simulink model "solarboat_solar"  (R2022a)
settings: Solver=VariableStepAuto  StartTime=0.0  StopTime=100  RelTol=1e-3
model workspace (MAT data in the model file):
  B = 0.67
  Cf = 0.00361699607356
  Dp = 0.2
  J = 1.6925
  K = 10
  KQ = 0.0168
  KT = 0.0514
  LOA = 1.8
  Re = 3577817.53131
  T = 1
  U = 5
  V_abs = 2
  d = 0.2
  mu = 1.188e-06
  psi_t = 0.174532925199
  rho = 1025
  weight = 8.036
  x_wp = 100
  y_wp = 100
libraries: fl_lib x12, nesl_utility x6, ee_lib x3, dspsrcs4 x2, slpidlib x1, spsPVArrayLib x1
settings Model: NumberOfSteps=100  Creator=takuya  LastModifiedBy=nakashima
settings OptimizationCC: ZeroExternalMemoryAtStartup=off  ZeroInternalMemoryAtStartup=off
settings DebuggingCC: UnconnectedInputMsg=warning  UnconnectedOutputMsg=warning  UnconnectedLineMsg=warning
settings RTWCC: TargetLang=C++  DLArmComputeVersion=19.05
settings GRTTargetCC: TargetLangStandard=C++11 (ISO)  CodeInterfacePackaging=C++ class

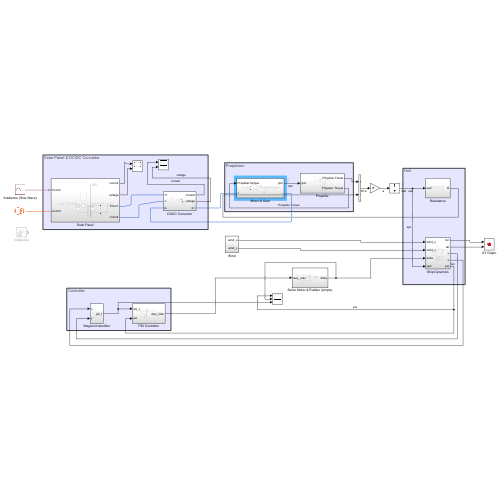
[thumbnail: Simulink's stored preview of the top-level diagram]
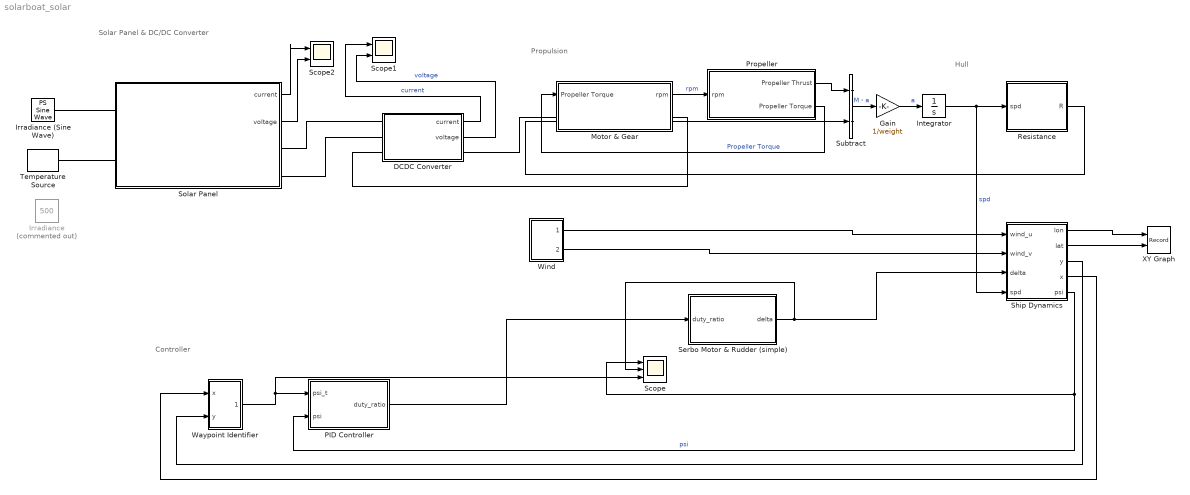
== system solarboat_solar ==
  note: Propulsion
  note: Solar Panel & DC/DC Converter
  note: Hull
  note: Controller
  DCDC Converter : Subsystem
  Gain : Gain  Gain=1/weight
  Integrator : Integrator
  Irradiance : Constant  Commented=on  Value=500
  Irradiance (Sine Wave) : fl_lib/Physical Signals/Sources/PS Sine Wave  amplitude=0 W/m^2  bias=500 W/m^2  frequency_spec=foundation.enum.frequencySpec.frequencySI  frequency_SI=0.1 Hz  frequency_angular=1 rad/s  phase=0 rad
      settings: SourceProductBaseCode=PW,SS,VE  InternalSimscapePortConfiguration="{\"Bottom\":[],\"Left\":[],\"Right\":[{\"id\":\"O\",\"label\":\"\",\"type\":\"output\"}],\"Top\":[]}"
  Motor & Gear : Subsystem
  PID Controller : Subsystem
  Propeller : Subsystem
  Resistance : Subsystem
  Scope : Scope  NumInputPorts=3
  Scope1 : Scope  NumInputPorts=2
  Scope2 : Scope  NumInputPorts=2
  Serbo Motor & Rudder (simple) : Subsystem
  Ship Dynamics : Subsystem
  Solar Panel : Subsystem
  Subtract : Sum  Inputs=+-
  Temperature Source : fl_lib/Thermal/Thermal Sources/Temperature Source  temperature=293.15 K
      settings: SourceProductBaseCode=PW,SS,VE
  Waypoint Identifier : Subsystem
  Wind : Subsystem
  XY Graph : Record  FileSettingsInternal="{\"entries\":[{\"content\":{\"excelSettings\":{\"content\":{},\"type\":\"Streamout.ExcelSettings\"}},\"type\":\"Streamout.FileSettingStorage\",\"uuid\":\"fc5eb300-97e0-4115-87c7-5fdc50d21362\"}],\"packageUris\":[\"http://schema.mathworks.com/mf0/streamout_blocks/R2020a\"],\"version\":\"1.0\"}"  Layout=[1 1]  SignalsInternal="{\"entries\":[{\"content\":{\"signals\":[{\"content\":{\"blockPath\":[\"solarboat_solar/XY Graph\"],\"channel\":[],\"dimensions\":[1],\"domain\":\"solarboat_solar/XY Graph\",\"lineColor\":\"#77ac30\",\"plots\":[],\"port\":1,\"sid\":[\"\"],\"signalID\":312,\"signalName\":\"Ship Dynamics:1\"},\"type\":\"RecordBlkView.Signal\",\"uuid\":\"acc7c85f-4951-4bf2-b97d-efe73aeb3011\"},{\"content\":{\"blockPath\":[\"solarboat_solar/XY Graph\"],\"channel\":[],\"dimensions\":[1],\"domain\":\"solarboat_solar/XY Graph\",\"lineColor\":\"#4dbeee\",\"plots\":[],\"port\":2,\"sid\":[\"\"],\"signalID\":316,\"signalName\":\"Ship Dynamics:2\"},\"type\":\"RecordBlkView.Signal\",\"uuid\":\"6ddd9926-56d6-4e91-80b1-5ee47d4dd409\"}]},\"type\":\"RecordBlkView.InputSignals\",\"uuid\":\"720abea7-f925-4eb8-95a6-226fe66648fe\"}],\"packageUris\":[\"http://schema.mathworks.com/mf0/streamout_blocks/R2020a\"],\"version\":\"1.0\"}"  VisualizationBindings="{\"xyplotplugin\":{\"info\":[{\"series\":[],\"subplotID\":1}]}}"  CompatibilityTag=XY  st=-1
  wires:
  Waypoint Identifier/1(psi_t) -> PID Controller/1(psi_t), Scope/3
  Subtract/1 -> Gain/1  "M・a"
  PID Controller/1(duty_ratio) -> Serbo Motor & Rudder (simple)/1(duty_ratio)
  Integrator/1 -> Ship Dynamics/4(spd), Resistance/1(spd)  "spd"
  Resistance/1(R) -> Subtract/2
  Ship Dynamics/1(lon) -> XY Graph/1
  Ship Dynamics/2(lat) -> XY Graph/2
  Ship Dynamics/4(x) -> Waypoint Identifier/1(x)
  Ship Dynamics/3(y) -> Waypoint Identifier/2(y)
  Serbo Motor & Rudder (simple)/1(delta) -> Ship Dynamics/3(delta), Scope/2
  Wind/1(wind_u) -> Ship Dynamics/1(wind_u)
  Ship Dynamics/5(psi) -> Scope/1, PID Controller/2(psi)  "psi"
  Wind/2(wind_v) -> Ship Dynamics/2(wind_v)
  Gain/1 -> Integrator/1  "a"
  DCDC Converter/1(current) -> Scope1/1  "current"
  DCDC Converter/2(voltage) -> Scope1/2  "voltage"
  Propeller/1(Propeller Thrust) -> Subtract/1
  Motor & Gear/1(rpm) -> Propeller/1(rpm)  "rpm"
  Propeller/2(Propeller Torque) -> Motor & Gear/1(Propeller Torque)  "Propeller Torque"
  Solar Panel/1(current) -> Scope2/1
  Solar Panel/2(voltage) -> Scope2/2
  connections:
  Motor & Gear/LConn1 -- DCDC Converter/RConn1
  DCDC Converter/LConn3 -- Motor & Gear/RConn1
  DCDC Converter/LConn1 -- Solar Panel/RConn1
  Irradiance (Sine Wave)/RConn1 -- Solar Panel/LConn1
  Solar Panel/LConn2 -- Temperature Source/LConn1
  Solar Panel/RConn2 -- DCDC Converter/LConn2

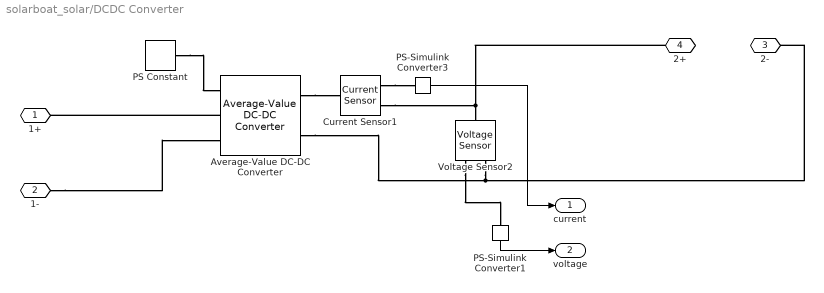
== system solarboat_solar/DCDC Converter ==
  Average-Value DC-DC Converter : ee_lib/Semiconductors & Converters/Converters/Average-Value DC-DC Converter  control_option=ee.enum.converters.controlinput.voltage  converter_type=ee.enum.converters.dcdctype.buck  efficiency_option=ee.enum.converters.efficiency.constant  efficiency_fixed=85  i_vec=[0, 2, 5] A  efficiency_vec=[90, 95, 98]
      settings: SourceProductBaseCode=PS  InternalSimscapePortConfiguration="{\"Bottom\":[],\"Left\":[{\"id\":\"Vref\",\"label\":\"Vref\",\"type\":\"input\"},{\"id\":\"p1\",\"label\":\"1+\",\"type\":\"foundation.electrical.electrical\"},{\"id\":\"n1\",\"label\":\"1-\",\"type\":\"foundation.electrical.electrical\"}],\"Right\":[{\"id\":\"p2\",\"label\":\"2+\",\"type\":\"foundation.electrical.electrical\"},{\"id\":\"n2\",\"label\":\"2-\",\"type\":\"foundation.electrical.electrical\"}],\"Top\":[]}"
  Current Sensor1 : fl_lib/Electrical/Electrical Sensors/Current Sensor
      settings: SourceProductBaseCode=PW,SS,VE
  PS Constant : fl_lib/Physical Signals/Sources/PS Constant  constant=12 V
      settings: SourceProductBaseCode=PW,SS,VE
  PS-Simulink Converter1 : nesl_utility/PS-Simulink Converter  PhysicalDomain=network_engine_domain  SubClassName=ps_output  LeftPortType=input  RightPortType=output  PseudoPeriodic=off  Frequencies=[]  VectorFormat=1-D array  Unit=inherit  AffineConversion=off
      settings: SourceProductBaseCode=SS,PW,VE
  PS-Simulink Converter3 : nesl_utility/PS-Simulink Converter  PhysicalDomain=network_engine_domain  SubClassName=ps_output  LeftPortType=input  RightPortType=output  PseudoPeriodic=off  Frequencies=[]  VectorFormat=1-D array  Unit=inherit  AffineConversion=off
      settings: SourceProductBaseCode=SS,PW,VE
  Voltage Sensor2 : fl_lib/Electrical/Electrical Sensors/Voltage Sensor
      settings: SourceProductBaseCode=PW,SS,VE
  1+ : PMIOPort  Side=Left
  1- : PMIOPort  Port=2  Side=Left
  2- : PMIOPort  Port=3  Side=Left
  2+ : PMIOPort  Port=4  Side=Right
  current : Outport
  voltage : Outport  Port=2
  wires:
  PS-Simulink Converter3/1 -> current/1
  PS-Simulink Converter1/1 -> voltage/1
  connections:
  PS Constant/RConn1 -- Average-Value DC-DC Converter/LConn1
  Average-Value DC-DC Converter/RConn2 -- 2-/RConn1 -- Voltage Sensor2/RConn2
  Current Sensor1/RConn2 -- 2+/RConn1 -- Voltage Sensor2/LConn1
  Voltage Sensor2/RConn1 -- PS-Simulink Converter1/LConn1
  Average-Value DC-DC Converter/RConn1 -- Current Sensor1/LConn1
  Current Sensor1/RConn1 -- PS-Simulink Converter3/LConn1
  Average-Value DC-DC Converter/LConn2 -- 1+/RConn1
  1-/RConn1 -- Average-Value DC-DC Converter/LConn3

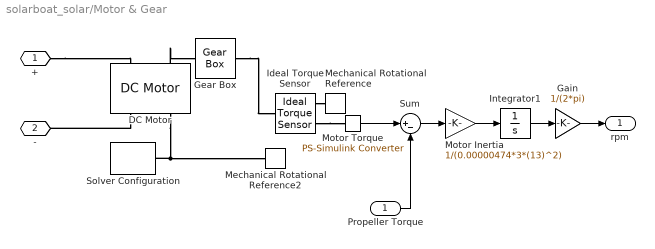
== system solarboat_solar/Motor & Gear ==
  Propeller Torque : Inport
  DC Motor : ee_lib/Electromechanical/Brushed Motors/DC Motor  field_option=ee.enum.field_option.pm  Rf=100 Ohm  Lf=1 H  Laf=0.15 H  If0=0 A  parameterization=ee.enum.dcparam_option.load_speed  Ra=3.9 Ohm  La=12e-6 H  emf_or_torque=ee.enum.emf_or_torque.kv  Kv=0.072e-3 V/rpm  Ki=6.876e-4 N*m/A  T_stall=0.24e-3 N*m  w_max=750*13 rpm  w_rated=750*11.1 rpm  P_rated=220 W  V_rated=11.1 V  lam_param=ee.enum.lam_param.current  i_noload=0.8 A  V_i_noload=13 V  J=0.00000474*3 kg*m^2  lam=0 N*m/(rad/s)  speed0=0 rpm  enable_fault_armature=simscape.enum.onoff.off  rev_faulted=1 / 3  G_faulted_armature=1e-5 S  fault_trigger_armature=ee.enum.faults.faultTrigger.temporal  t_fault_armature=1 s  max_permissible_current_armature=inf A  t_fail_on_current_armature=1 s  enable_fault_field=simscape.enum.onoff.off  G_faulted_field=1e-5 S  fault_trigger_field=ee.enum.faults.faultTrigger.temporal  t_fault_field=1 s  max_permissible_current_field=inf A  t_fail_on_current_field=1 s  fault_action=simscape.enum.assert.action.none  alpha=3.93e-3 1/K  Tmeas=25 degC  thermal_mass=100 J/K  initial_temperature=25 degC
  Gain : Gain  Gain=1/(2*pi)
  Gear Box : fl_lib/Mechanical/Mechanisms/Gear Box  ratio=13  t_in_specify=off  t_in_priority=None  t_in=0 N*m  t_in_nominal_specify=off  t_in_nominal_unit=N*m  t_in_nominal_value=1  t_out_specify=off  t_out_priority=None  t_out=0 N*m  t_out_nominal_specify=off  t_out_nominal_unit=N*m  t_out_nominal_value=1
      settings: SourceProductBaseCode=PW,SS,VE
  Ideal Torque Sensor : fl_lib/Mechanical/Mechanical Sensors/Ideal Torque Sensor
      settings: SourceProductBaseCode=PW,SS,VE
  Integrator1 : Integrator
  Mechanical Rotational Reference : fl_lib/Mechanical/Rotational Elements/Mechanical Rotational Reference
      settings: SourceProductBaseCode=PW,SS,VE
  Mechanical Rotational Reference2 : fl_lib/Mechanical/Rotational Elements/Mechanical Rotational Reference
      settings: SourceProductBaseCode=PW,SS,VE
  Motor Inertia : Gain  Gain=1/(0.00000474*3*(13)^2)
  Motor Torque : nesl_utility/PS-Simulink Converter  PhysicalDomain=network_engine_domain  SubClassName=ps_output  LeftPortType=input  RightPortType=output  PseudoPeriodic=off  Frequencies=[]  VectorFormat=1-D array  Unit=inherit  AffineConversion=off
      settings: SourceProductBaseCode=SS,PW,VE
  Solver Configuration : nesl_utility/Solver Configuration  PhysicalDomain=network_engine_domain  SubClassName=solver  LeftPortType=input  RightPortType=generic  Tones=[]  Harmonics=[]  SimulateNoise=off  Profile=off  UseLocalSampling=off  EnableSwitchedLinearOptims=on  FrequencyDomain=off  UseCCode=off  RelTol=0.001  AbsTol=1e-06  MinStep=1e-09  ToWorkspace=off  RevertToSquareIcSolve=off  NumHomotopyIterations=100  PhasorMode=off  PhasorModeNumHarmonics=1  IndexReductionMethod=DerivativeReplacement  DoDC=off  ResidualTolerance=1e-09  UseLocalSolver=off  LocalSolverChoice=NE_BACKWARD_EULER_ADVANCER  LocalSolverSampleTime=0.001  DoFixedCost=off  MaxNonlinIter=3  MaxModeIter=2  ComputeImpulses=off  ImpulseIterations=2  LinearAlgebra=auto  LinearAlgebraNumThread=0  EquationFormulation=NE_TIME_EF  DelaysMemoryBudget=1024  AutomaticFiltering=on  FilteringTimeConstant=0.001  PartitionStorageMethod=AS_NEEDED  PartitionMemoryBudget=1024  PartitionMethod=ROBUST
      settings: SourceProductBaseCode=SS,PW,VE
  Sum : Sum  Inputs=|+-
  + : PMIOPort  Side=Left
  - : PMIOPort  Port=2  Side=Right
  rpm : Outport
  wires:
  Gain/1 -> rpm/1
  Integrator1/1 -> Gain/1
  Sum/1 -> Motor Inertia/1
  Motor Torque/1 -> Sum/1
  Motor Inertia/1 -> Integrator1/1
  Propeller Torque/1 -> Sum/2
  connections:
  Ideal Torque Sensor/RConn1 -- Mechanical Rotational Reference/LConn1
  DC Motor/LConn2 -- Gear Box/LConn1
  DC Motor/RConn2 -- Mechanical Rotational Reference2/LConn1 -- Solver Configuration/RConn1
  +/RConn1 -- DC Motor/LConn1
  Ideal Torque Sensor/RConn2 -- Motor Torque/LConn1
  Gear Box/RConn1 -- Ideal Torque Sensor/LConn1
  DC Motor/RConn1 -- -/RConn1

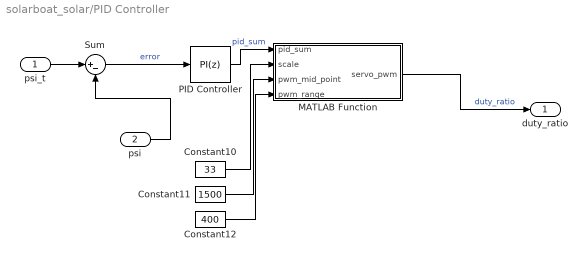
== system solarboat_solar/PID Controller ==
  psi_t : Inport
  psi : Inport  Port=2
  Constant10 : Constant  Value=33
  Constant11 : Constant  Value=1500
  Constant12 : Constant  Value=400
  MATLAB Function : MATLAB Function  TreatAsAtomicUnit=on
  PID Controller : slpidlib/PID Controller  Controller=PI  Form=Parallel  TimeDomain=Discrete-time  UseExternalTs=off  SampleTime=1  IntegratorMethod=Forward Euler  FilterMethod=Forward Euler  ControllerParametersSource=internal  P=10  I=1  UseKiTs=off  D=0  N=0.125  UseFilter=on  TunerSelectOption=Transfer Function Based (PID Tuner App)  ZeroCross=off  InitialConditionSource=internal  InitialConditionForIntegrator=0  InitialConditionForFilter=0  DifferentiatorICPrevScaledInput=0  ExternalReset=none  TrackingMode=off  Kt=1  LimitOutput=off  SatLimitsSource=internal  UpperSaturationLimit=inf  LowerSaturationLimit=-inf  LinearizeAsGain=on  AntiWindupMode=none  Kb=1  POutMin=[]  POutMax=[]  IOutMin=[]  IOutMax=[]  DOutMin=[]  DOutMax=[]  NOutMin=[]  NOutMax=[]  SumOutMin=[]  SumOutMax=[]  SaturationOutMin=[]  SaturationOutMax=[]  PParamMin=[]  PParamMax=[]  IParamMin=[]  IParamMax=[]  DParamMin=[]  DParamMax=[]  NParamMin=[]  NParamMax=[]  KbParamMin=[]  KbParamMax=[]  KtParamMin=[]  KtParamMax=[]  KbOutMin=[]  KbOutMax=[]  KtOutMin=[]  KtOutMax=[]  IntegratorOutMin=[]  IntegratorOutMax=[]  FilterOutMin=[]  FilterOutMax=[]  SumI1OutMin=[]  SumI1OutMax=[]  SumI2OutMin=[]  SumI2OutMax=[]  SumI3OutMin=[]  SumI3OutMax=[]  SumI4OutMin=[]  SumI4OutMax=[]  SumDOutMin=[]  SumDOutMax=[]  DifferentiatorOutMin=[]  DifferentiatorOutMax=[]  FilterDiffOutCoefMin=[]  FilterDiffOutCoefMax=[]  ReciprocalOutMin=[]  ReciprocalOutMax=[]  SumDenOutMin=[]  SumDenOutMax=[]  SumNumOutMin=[]  SumNumOutMax=[]  DivideOutMin=[]  DivideOutMax=[]  UdiffTsProdOutMin=[]  UdiffTsProdOutMax=[]  NTsProdOutMin=[]  NTsProdOutMax=[]  UintegralTsProdOutMin=[]  UintegralTsProdOutMax=[]  UngainTsProdOutMin=[]  UngainTsProdOutMax=[]  IntegratorContinuousStateAttributes=''  IntegratorStateMustResolveToSignalObject=off  IntegratorRTWStateStorageClass=Auto  FilterContinuousStateAttributes=''  FilterStateMustResolveToSignalObject=off  FilterRTWStateStorageClass=Auto  ParallelPVariant=InternalParameters  IdealPVariant=Disabled  IVariant=InternalParameters  DVariant=Disabled  IntegratorVariant=Discrete  SatVariant=Disabled  AWVariant=Passthrough  PCopyVariant=Disabled  TRVariant=Disabled  FdbkBlocksVariant=Forward  IdealPFdbkVariant=Disabled  SatFdbkVariant=Disabled  DerivativeFilterVariant=Disabled  NVariant=Disabled  NCopyVariant=Disabled_SignalSpec  FilterICVariant=Disabled  IntegratorICVariant=InternalICs  ExternalResetVariant=Disabled  TRSumVariant=Passthrough  SumFdbkVariant=Disabled  SumVariant=Sum_PI  TsampFilterVariant=InternalTs  TsampNgainVariant=Passthrough  TsampIntegralVariant=Passthrough  ExternalSaturationOutDataTypeStr=Inherit: Same as second input  aMode=0
  Sum : Sum  Inputs=|+-
  duty_ratio : Outport
  wires:
  psi/1 -> Sum/2
  Constant11/1 -> MATLAB Function/3(pwm_mid_point)
  psi_t/1 -> Sum/1
  Constant12/1 -> MATLAB Function/4(pwm_range)
  PID Controller/1 -> MATLAB Function/1(pid_sum)  "pid_sum"
  MATLAB Function/1(servo_pwm) -> duty_ratio/1  "duty_ratio"
  Sum/1 -> PID Controller/1  "error"
  Constant10/1 -> MATLAB Function/2(scale)

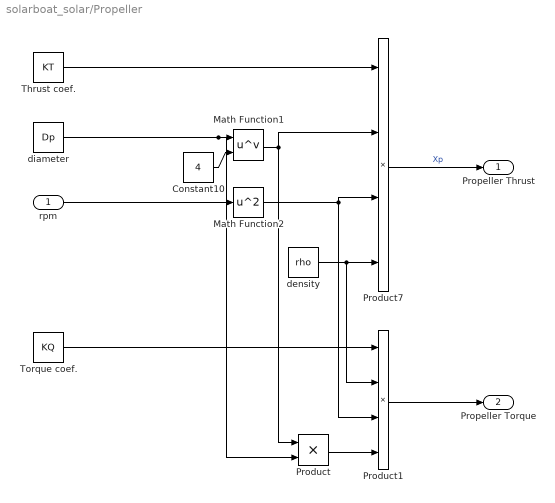
== system solarboat_solar/Propeller ==
  rpm : Inport
  Constant10 : Constant  Value=4
  Math Function1 : Math  Operator=pow
  Math Function2 : Math  Operator=square
  Product : Product
  Product1 : Product  Inputs=4
  Product7 : Product  Inputs=4
  Thrust coef. : Constant  Value=KT
  Torque coef. : Constant  Value=KQ
  density : Constant  Value=rho
  diameter : Constant  Value=Dp
  Propeller Thrust : Outport
  Propeller Torque : Outport  Port=2
  wires:
  diameter/1 -> Product/2, Math Function1/1
  Constant10/1 -> Math Function1/2
  Math Function2/1 -> Product1/3, Product7/3
  Thrust coef./1 -> Product7/1
  Math Function1/1 -> Product/1, Product7/2
  density/1 -> Product7/4, Product1/2
  rpm/1 -> Math Function2/1
  Product7/1 -> Propeller Thrust/1  "Xp"
  Torque coef./1 -> Product1/1
  Product/1 -> Product1/4
  Product1/1 -> Propeller Torque/1

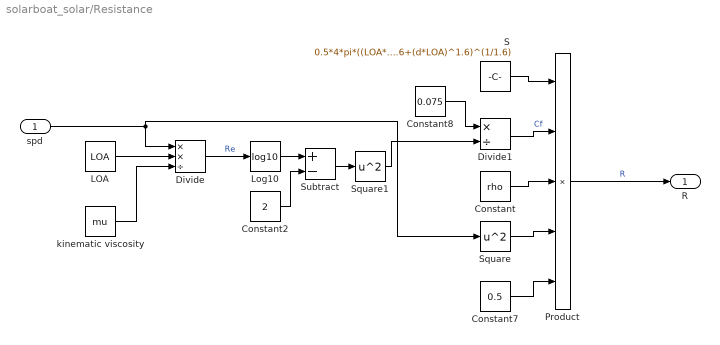
== system solarboat_solar/Resistance ==
  spd : Inport
  Constant : Constant  Value=rho
  Constant2 : Constant  Value=2
  Constant7 : Constant  Value=0.5
  Constant8 : Constant  Value=0.075
  Divide : Product  Inputs=**/
  Divide1 : Product  Inputs=*/
  LOA : Constant  Value=LOA
  Log10 : Math  Operator=log10
  Product : Product  Inputs=5
  S : Constant  Value=0.5*4*pi*((LOA*B)^1.6+(B*d)^1.6+(d*LOA)^1.6)^(1/1.6)
  Square : Math  Operator=square
  Square1 : Math  Operator=square
  Subtract : Sum  Inputs=+-
  kinematic viscosity : Constant  Value=mu
  R : Outport
  wires:
  spd/1 -> Square/1, Divide/1
  Square/1 -> Product/4
  Constant7/1 -> Product/5
  LOA/1 -> Divide/2
  Constant/1 -> Product/3
  Constant2/1 -> Subtract/2
  kinematic viscosity/1 -> Divide/3
  Divide/1 -> Log10/1  "Re"
  S/1 -> Product/1
  Divide1/1 -> Product/2  "Cf"
  Square1/1 -> Divide1/2
  Product/1 -> R/1  "R"
  Log10/1 -> Subtract/1
  Constant8/1 -> Divide1/1
  Subtract/1 -> Square1/1

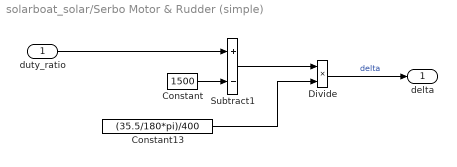
== system solarboat_solar/Serbo Motor & Rudder (simple) ==
  duty_ratio : Inport
  Constant : Constant  Value=1500
  Constant13 : Constant  Value=(35.5/180*pi)/400
  Divide : Product  Inputs=**
  Subtract1 : Sum  Inputs=+-
  delta : Outport
  wires:
  Subtract1/1 -> Divide/1
  Constant/1 -> Subtract1/2
  Constant13/1 -> Divide/2
  duty_ratio/1 -> Subtract1/1
  Divide/1 -> delta/1  "delta"

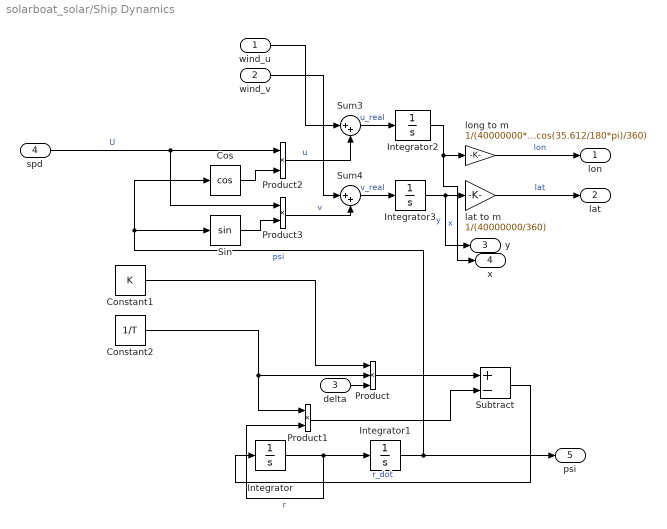
== system solarboat_solar/Ship Dynamics ==
  wind_u : Inport
  wind_v : Inport  Port=2
  delta : Inport  Port=3
  spd : Inport  Port=4
  Constant1 : Constant  Value=K
  Constant2 : Constant  Value=1/T
  Cos : Trigonometry  Operator=cos
  Integrator : Integrator
  Integrator1 : Integrator
  Integrator2 : Integrator  InitialCondition=139.18811*40000000*cos(35.612/180*pi)/360
  Integrator3 : Integrator  InitialCondition=35.61204*40000000/360
  Product : Product  Inputs=3
  Product1 : Product
  Product2 : Product
  Product3 : Product
  Sin : Trigonometry
  Subtract : Sum  Inputs=+-
  Sum3 : Sum  Inputs=|++
  Sum4 : Sum  Inputs=|++
  lat to m : Gain  Gain=1/(40000000/360)
  long to m : Gain  Gain=1/(40000000*cos(35.612/180*pi)/360)
  lon : Outport
  lat : Outport  Port=2
  y : Outport  Port=3
  x : Outport  Port=4
  psi : Outport  Port=5
  wires:
  Product1/1 -> Subtract/2
  wind_v/1 -> Sum4/1
  Integrator/1 -> Integrator1/1, Product1/2  "r"
  Integrator2/1 -> x/1, long to m/1  "x"
  Constant1/1 -> Product/1
  Sum4/1 -> Integrator3/1  "v_real"
  Product/1 -> Subtract/1
  Product3/1 -> Sum4/2  "v"
  Product2/1 -> Sum3/2  "u"
  Cos/1 -> Product2/2
  Sin/1 -> Product3/2
  Integrator3/1 -> y/1, lat to m/1  "y"
  Integrator1/1 -> Cos/1, Sin/1, psi/1  "psi"
  Subtract/1 -> Integrator/1  "r_dot"
  spd/1 -> Product3/1, Product2/1  "U"
  Constant2/1 -> Product1/1, Product/2
  Sum3/1 -> Integrator2/1  "u_real"
  wind_u/1 -> Sum3/1
  delta/1 -> Product/3
  long to m/1 -> lon/1  "lon"
  lat to m/1 -> lat/1  "lat"

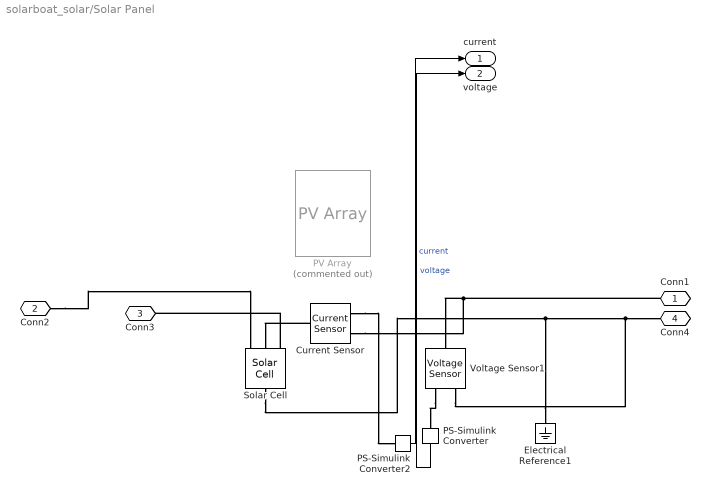
== system solarboat_solar/Solar Panel ==
  Current Sensor : fl_lib/Electrical/Electrical Sensors/Current Sensor
      settings: SourceProductBaseCode=PW,SS,VE
  Electrical Reference1 : fl_lib/Electrical/Electrical Elements/Electrical Reference
      settings: SourceProductBaseCode=PW,SS,VE
  PS-Simulink Converter : nesl_utility/PS-Simulink Converter  PhysicalDomain=network_engine_domain  SubClassName=ps_output  LeftPortType=input  RightPortType=output  PseudoPeriodic=off  Frequencies=[]  VectorFormat=1-D array  Unit=inherit  AffineConversion=off
      settings: SourceProductBaseCode=SS,PW,VE
  PS-Simulink Converter2 : nesl_utility/PS-Simulink Converter  PhysicalDomain=network_engine_domain  SubClassName=ps_output  LeftPortType=input  RightPortType=output  PseudoPeriodic=off  Frequencies=[]  VectorFormat=1-D array  Unit=inherit  AffineConversion=off
      settings: SourceProductBaseCode=SS,PW,VE
  PV Array : spsPVArrayLib/PV Array  Commented=on  Npar=40  Nser=10  PlotType=array @ 1000 W/m2 & specified temperatures  S_vec="[ 1000  500  100 ]"  Temp_C_vec="[ 45 25  ]"  ModuleName=User-defined  PlotWhenSelected=off  Pm=213.15  Ncell=60  Voc=36.3  Isc=7.84  Vm=29  Im=7.35  beta_Voc_pc=-0.36099  alpha_Isc_pc=0.102  beta_Voc=-0.13104  alpha_Isc=0.0079968  IL=7.8654  I0=2.9273e-10  nI=0.98119  Rsh=313.0553  Rs=0.39381  RobustModel=off  RobustCellTemperature=313.3991  BAL=on  Tc=1e-6  Tfilter=5e-5
  Solar Cell : ee_lib/Sources/Solar Cell  prm=1  Isc=9.5 A  Voc=23.9 V  Is=1e-6 A  Is2=0 A  Iph=7.34 A  Ir0=1000 W/m^2  ec=1.5  N2=2  Rs=1 Ohm  Rp=inf Ohm  N_series=4  N_parallel=9  TIPH1=0.005 1/K  EG=1.11 eV  TXIS1=3  TXIS2=3  TRS1=0  TRP1=0  Tmeas=25 degC  TFIXED=25 degC  thermal_mass=100 J/K  initial_temperature=25 degC
      settings: SourceProductBaseCode=PS  InternalSimscapePortConfiguration="{\"Bottom\":[],\"Left\":[{\"id\":\"Ir\",\"label\":\"Ir\",\"type\":\"input\"},{\"id\":\"p\",\"label\":\"+\",\"type\":\"foundation.electrical.electrical\"},{\"id\":\"H\",\"label\":\"H\",\"type\":\"foundation.thermal.thermal\"}],\"Right\":[{\"id\":\"n\",\"label\":\"-\",\"type\":\"foundation.electrical.electrical\"}],\"Top\":[]}"
  Voltage Sensor1 : fl_lib/Electrical/Electrical Sensors/Voltage Sensor
      settings: SourceProductBaseCode=PW,SS,VE
  Conn1 : PMIOPort  Side=Right
  Conn2 : PMIOPort  Port=2  Side=Left
  Conn3 : PMIOPort  Port=3  Side=Left
  Conn4 : PMIOPort  Port=4  Side=Right
  current : Outport
  voltage : Outport  Port=2
  wires:
  PS-Simulink Converter/1 -> voltage/1  "voltage"
  PS-Simulink Converter2/1 -> current/1  "current"
  connections:
  Current Sensor/RConn2 -- Conn1/RConn1 -- Voltage Sensor1/LConn1
  Voltage Sensor1/RConn1 -- PS-Simulink Converter/LConn1
  Current Sensor/LConn1 -- Solar Cell/LConn2
  Current Sensor/RConn1 -- PS-Simulink Converter2/LConn1
  Electrical Reference1/LConn1 -- Solar Cell/RConn1 -- Conn4/RConn1 -- Voltage Sensor1/RConn2
  Solar Cell/LConn3 -- Conn3/RConn1
  Conn2/RConn1 -- Solar Cell/LConn1

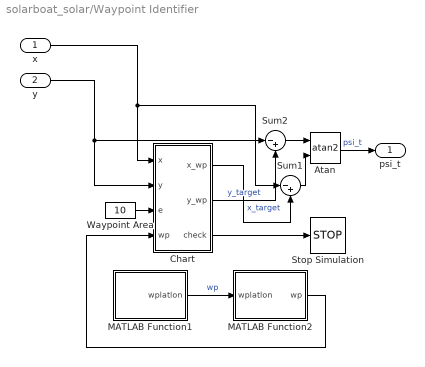
== system solarboat_solar/Waypoint Identifier ==
  x : Inport
  y : Inport  Port=2
  Atan : Trigonometry  Operator=atan2
  Chart : Stateflow chart  TreatAsAtomicUnit=on
  MATLAB Function1 : MATLAB Function  TreatAsAtomicUnit=on
  MATLAB Function2 : MATLAB Function  TreatAsAtomicUnit=on
  Stop Simulation : Stop
  Sum1 : Sum  Inputs=|-+
  Sum2 : Sum  Inputs=|-+
  Waypoint Area : Constant  Value=10
  psi_t : Outport
  wires:
  Chart/3(check) -> Stop Simulation/1
  Sum1/1 -> Atan/2
  Waypoint Area/1 -> Chart/3(e)
  x/1 -> Sum1/1, Chart/1(x)
  y/1 -> Chart/2(y), Sum2/1
  Sum2/1 -> Atan/1
  Chart/1(x_wp) -> Sum1/2  "x_target"
  MATLAB Function2/1(wp) -> Chart/4(wp)
  Chart/2(y_wp) -> Sum2/2  "y_target"
  MATLAB Function1/1(wplatlon) -> MATLAB Function2/1(wplatlon)  "wp"
  Atan/1 -> psi_t/1  "psi_t"

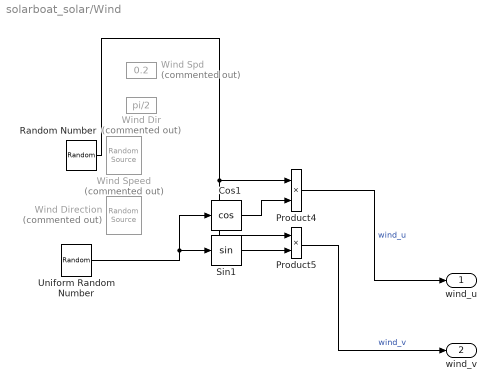
== system solarboat_solar/Wind ==
  Cos1 : Trigonometry  Operator=cos
  Product4 : Product
  Product5 : Product
  Random Number : RandomNumber  SampleTime=0.1
  Sin1 : Trigonometry
  Uniform Random Number : UniformRandomNumber  Minimum=0  Maximum=2*pi  SampleTime=0.1
  Wind Dir : Constant  Commented=on  Value=pi/2
  Wind Direction : dspsrcs4/Random Source  Commented=on  SrcType=Uniform  NormMethod=Ziggurat  CltLength=12  MinVal=0  MaxVal=2*pi  MeanVal=0  VarVal=1  RepMode=Not repeatable  rawSeed=1  IsInherit=off  SampMode=Discrete  SampTime=1  SampFrame=1  DataType=Double  OutComplex=Real  OutputFrames=off
  Wind Spd : Constant  Commented=on  Value=0.2
  Wind Speed : dspsrcs4/Random Source  Commented=on  SrcType=Uniform  NormMethod=Ziggurat  CltLength=12  MinVal=0  MaxVal=0.5  MeanVal=0  VarVal=1  RepMode=Not repeatable  rawSeed=1  IsInherit=off  SampMode=Discrete  SampTime=1  SampFrame=1  DataType=Double  OutComplex=Real  OutputFrames=off
  wind_u : Outport
  wind_v : Outport  Port=2
  wires:
  Random Number/1 -> Product5/1, Product4/1
  Cos1/1 -> Product4/2
  Uniform Random Number/1 -> Cos1/1, Sin1/1
  Sin1/1 -> Product5/2
  Product5/1 -> wind_v/1  "wind_v"
  Product4/1 -> wind_u/1  "wind_u"

== matlab function solarboat_solar/Waypoint Identifier/MATLAB Function1 ==
  data: wplatlon output
function wplatlon = ReadWP()
coder.extrinsic('readmatrix');
wp = zeros(6,2);
wp = readmatrix('wp_test_210803.txt');
wplatlon = flip(wp,2)

== matlab function solarboat_solar/PID Controller/MATLAB Function ==
  data: pid_sum input; servo_pwm output; scale input; pwm_mid_point input; pwm_range input
function servo_pwm = fcn(pid_sum,scale,pwm_mid_point,pwm_range)
temp = exp(-pid_sum / scale)
pid_sum_norm = (2 / (1 + temp)) - 1
servo_pwm = pwm_mid_point + pwm_range * pid_sum_norm

== stateflow chart solarboat_solar/Waypoint Identifier/Chart ==
  state waypoint1
    entry:
    x_wp = wp(1,1);
    y_wp = wp(1,2);
    n=1
    check = 0
  state waypointn
    entry:
    n=n+1
    if n <= numel(wp)/2
    x_wp = wp(n,1);
    y_wp = wp(n,2);
    end
  state end
    entry:
    check = 1
  (default) -> waypoint1
  waypoint1 -> waypointn : [x >= wp(1,1) && x < wp(1,1)+e && y >=wp(1,2) && y < wp(1,2) +e]
  waypointn -> waypointn [order 2] : [x >= wp(n,1) && x < wp(n,1)+e && y >=wp(n,2) && y < wp(n,2) +e]
  waypointn -> end [order 1] : [n > numel(wp)/2]
  data: x input; y input; x_wp output; y_wp output; e input; n local; check output; wp input

== matlab function solarboat_solar/Waypoint Identifier/MATLAB Function2 ==
  data: wplatlon input; wp output
function wp = wp_t(wplatlon)
wp=zeros(size(wplatlon))
wp(:,1)=wplatlon(:,1)*40000000*cos(35.612/180*pi)/360
wp(:,2)=wplatlon(:,2)*40000000/360
